simulink model "Controller"  (R2018b)
settings: configuration reference "FixedStepConfiguration" (kept outside this file)
settings Model: DataDictionary=DataDictionary.sldd  Creator=chris  LastModifiedBy=chris

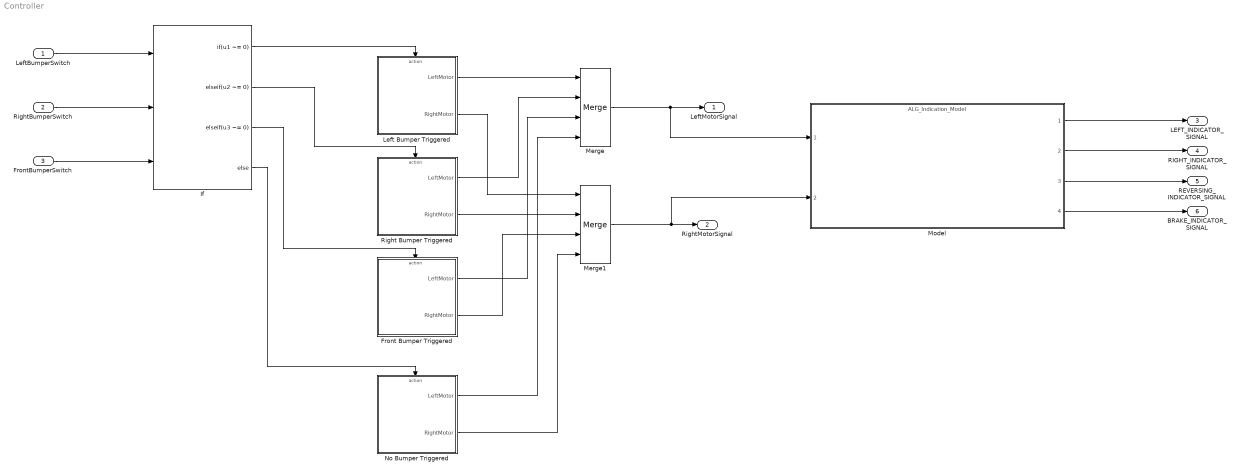
== system Controller ==
  LeftBumperSwitch : Inport
  RightBumperSwitch : Inport  Port=2
  FrontBumperSwitch : Inport  Port=3
  Front Bumper Triggered : Subsystem
  If : If  NumInputs=3  IfExpression=u1 ~= 0  ElseIfExpressions=u2 ~= 0, u3 ~= 0
  Left Bumper Triggered : Subsystem
  Merge : Merge  Inputs=4
  Merge1 : Merge  Inputs=4
  Model : ModelReference  ModelNameDialog=ALG_Indication_Model.slx  SimulationMode=Normal  ModelReferenceVersion=1.3
  No Bumper Triggered : Subsystem
  Right Bumper Triggered : Subsystem
  "LeftMotorSignal " : Outport
  RightMotorSignal : Outport  Port=2
  LEFT_INDICATOR_SIGNAL : Outport  Port=3
  RIGHT_INDICATOR_SIGNAL : Outport  Port=4
  REVERSING_INDICATOR_SIGNAL : Outport  Port=5
  BRAKE_INDICATOR_SIGNAL : Outport  Port=6
  wires:
  LeftBumperSwitch/1 -> If/1
  RightBumperSwitch/1 -> If/2
  FrontBumperSwitch/1 -> If/3
  If/1 -> Left Bumper Triggered/Action
  Merge/1 -> Model/1, "LeftMotorSignal "/1
  Left Bumper Triggered/1(LeftMotor) -> Merge/1
  Right Bumper Triggered/1(LeftMotor) -> Merge/2
  Front Bumper Triggered/1(LeftMotor) -> Merge/3
  No Bumper Triggered/1(LeftMotor) -> Merge/4
  Merge1/1 -> Model/2, RightMotorSignal/1
  Left Bumper Triggered/2(RightMotor) -> Merge1/1
  Right Bumper Triggered/2(RightMotor) -> Merge1/2
  Front Bumper Triggered/2(RightMotor) -> Merge1/3
  No Bumper Triggered/2(RightMotor) -> Merge1/4
  If/2 -> Right Bumper Triggered/Action
  If/3 -> Front Bumper Triggered/Action
  If/4 -> No Bumper Triggered/Action
  Model/1 -> LEFT_INDICATOR_SIGNAL/1
  Model/2 -> RIGHT_INDICATOR_SIGNAL/1
  Model/3 -> REVERSING_INDICATOR_SIGNAL/1
  Model/4 -> BRAKE_INDICATOR_SIGNAL/1

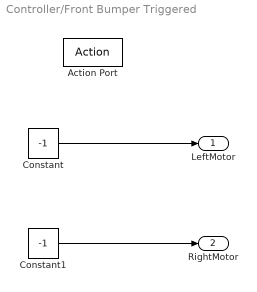
== system Controller/Front Bumper Triggered ==
  Action Port : ActionPort  ActionType=elseif
  Constant : Constant  Value=-1
  Constant1 : Constant  Value=-1
  LeftMotor : Outport
  RightMotor : Outport  Port=2
  wires:
  Constant/1 -> LeftMotor/1
  Constant1/1 -> RightMotor/1

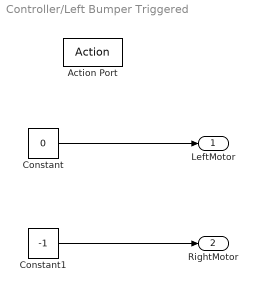
== system Controller/Left Bumper Triggered ==
  Action Port : ActionPort  ActionType=then
  Constant : Constant  Value=0
  Constant1 : Constant  Value=-1
  LeftMotor : Outport
  RightMotor : Outport  Port=2
  wires:
  Constant/1 -> LeftMotor/1
  Constant1/1 -> RightMotor/1

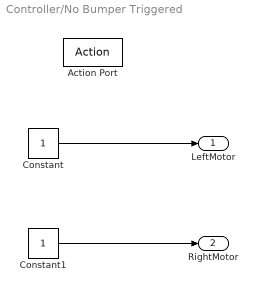
== system Controller/No Bumper Triggered ==
  Action Port : ActionPort  ActionType=else
  Constant : Constant
  Constant1 : Constant
  LeftMotor : Outport
  RightMotor : Outport  Port=2
  wires:
  Constant1/1 -> RightMotor/1
  Constant/1 -> LeftMotor/1

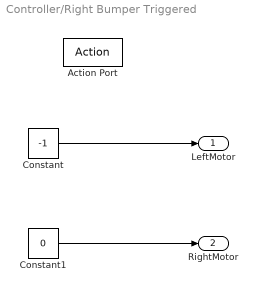
== system Controller/Right Bumper Triggered ==
  Action Port : ActionPort  ActionType=elseif
  Constant : Constant  Value=-1
  Constant1 : Constant  Value=0
  LeftMotor : Outport
  RightMotor : Outport  Port=2
  wires:
  Constant1/1 -> RightMotor/1
  Constant/1 -> LeftMotor/1
